simulink model "PI_tacho"  (R2019b)
settings: Solver=VariableStepAuto  StartTime=0.0  StopTime=80  RelTol=1e-3
values from neighbouring files (symbols this model uses):
  kd = 4    [skrypt.m]
  ki = 3    [skrypt.m]
  kp = 2    [skrypt.m]
settings Model: Creator=szymo  LastModifiedBy=szymo

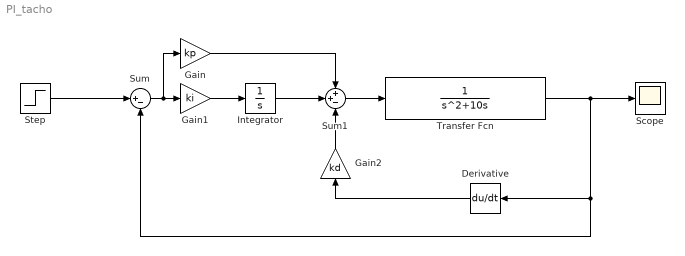
== system PI_tacho ==
  Derivative : Derivative
  Gain : Gain  Gain=kp
  Gain1 : Gain  Gain=ki
  Gain2 : Gain  Gain=kd
  Integrator : Integrator
  Scope : Scope
  Step : Step  Time=0  SampleTime=0
  Sum : Sum  Inputs=|+-
  Sum1 : Sum  Inputs=++-
  Transfer Fcn : TransferFcn  Denominator=[1 10 0]
  wires:
  Step/1 -> Sum/1
  Integrator/1 -> Sum1/2
  Sum/1 -> Gain/1, Gain1/1
  Gain1/1 -> Integrator/1
  Gain/1 -> Sum1/1
  Sum1/1 -> Transfer Fcn/1
  Transfer Fcn/1 -> Sum/2, Derivative/1, Scope/1
  Derivative/1 -> Gain2/1
  Gain2/1 -> Sum1/3
